simulink model "rtMotomanVR_vaja7"  (R2019b)
settings: Solver=FixedStepDiscrete  StartTime=0.0  StopTime=30  FixedStep=dT  RelTol=1e-3  EnableMultiTasking=on
values from neighbouring files (symbols this model uses):
  dT = 1/500    (= 0.002)    [initVR.m]    (also in trajectory.m = 0.00025)
  fbGain = 20    [initVR.m]    (also in trajectory.m)
  q0 = [0 0 0 0 90 0]'*pi/180    [initVR.m]    (also in trajectory.m)
undefined symbols (not defined in the file or in its folder): DiscIntNeverNeededParam, q2ZYXeul
libraries: simulink x2, xpcutilitieslib x2, dspnetwork x2, dspinverses x1
Description:
  | Real-Time Van der Pol Simulation
  | 
  | This demonstration shows a real-time version of the Simulink Van der Pol
  | simulation demo. This model does not need any external signals, so it does
  | not need any data acquisition hardware or driver. This makes the model ideal
  | for first experiments with Real-Time Windows Target, without need to
  | worry about proper I/O hardware configuration.
  | 
  | How to run this demo:
  | 
  |   1. Build the model using Tools -> Real-Time Workshop -> Build Model.
  |   2. Connect to the real-time code using Simulation -> Connect to target.
  |   3. Start the real-time execution using Simulation -> Start real-time code.
settings Model: EnablePacing=on  Creator=Houska  LastModifiedBy=student
settings DataIOCC: LimitDataPoints=on  SaveFormat=Array  SignalLoggingSaveFormat=ModelDataLogs  SaveOutput=off  SaveTime=off  ReturnWorkspaceOutputs=off  SignalLoggingName=logsOut
settings OptimizationCC: ExpressionDepthLimit=2147483647  InitFltsAndDblsToZero=on  LifeSpan=inf
settings DebuggingCC: SaveWithParameterizedLinksMsg=none  UnderspecifiedInitializationDetection=Classic  MergeDetectMultiDrivingBlocksExec=none  SignalResolutionControl=TryResolveAllWithWarning  MultiTaskDSMMsg=warning  MultiTaskCondExecSysMsg=none  FcnCallInpInsideContextMsg=warning  StateNameClashWarn=warning  SFUnexpectedBacktrackingDiag=warning  SFNoUnconditionalDefaultTransitionDiag=warning  SFExecutionAtInitializationDiag=none  ArithmeticOperatorsInVariantConditions=warning
settings HardwareCC: ProdBitPerPointer=32  ProdBitPerSizeT=32  ProdBitPerPtrDiffT=32  ProdLargestAtomicFloat=None  ProdWordSize=32  ProdHWDeviceType=32-bit Real-Time Windows Target
settings ModelReferenceCC: PropagateSignalLabelsOutOfModel=off
settings SFSimCC: SimUseLocalCustomCode=off  SimParseCustomCode=off  CustomCodeUndefinedFunction=UseInterfaceOnly
settings RTWCC: Description=Real-Time Windows Target  SystemTargetFile=rtwin.tlc  TemplateMakefile=rtwin.tmf  RTWUseLocalCustomCode=off
settings CodeAppCC: StateflowObjectComments=on
settings TargetCC: TargetFcnLib=ansi_tfl_tmw.mat  ModelReferenceCompliant=off  CompOptLevelCompliant=off  PreserveStateflowLocalDataDimensions=off
settings ConfigComp: CovMetricSettings=dw  CovHtmlReporting=on  CovSaveCumulativeToWorkspaceVar=on  CovSaveSingleToWorkspaceVar=on  CovExternalEMLEnable=off

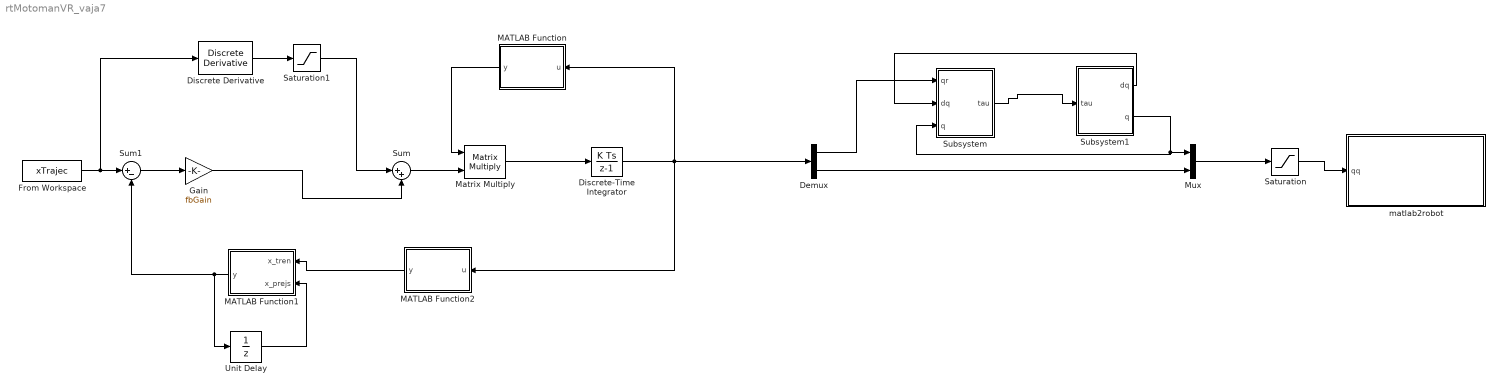
== system rtMotomanVR_vaja7 ==
  Demux : Demux  Outputs=2
  Discrete Derivative : simulink/Discrete/Discrete Derivative  gainval=1.0  ICPrevScaledInput=0.0  OutMin=[]  OutMax=[]  OutDataType=fixdt(1, 16)  OutScaling=2^-10  DoSatur=off
  Discrete-Time Integrator : DiscreteIntegrator  InitialCondition=q0  SampleTime=dT  ICPrevOutput=DiscIntNeverNeededParam  ICPrevScaledInput=DiscIntNeverNeededParam
  From Workspace : FromWorkspace  VariableName=xTrajec  SampleTime=0
  Gain : Gain  Gain=fbGain
  MATLAB Function : MATLAB Function  TreatAsAtomicUnit=on
  MATLAB Function1 : MATLAB Function  TreatAsAtomicUnit=on
  MATLAB Function2 : MATLAB Function  TreatAsAtomicUnit=on
  Matrix Multiply : Product  Multiplication=Matrix(*)
  Mux : Mux  Inputs=2
  Saturation : Saturate  UpperLimit=([94.5, 75, 45, 160, 120 180]-5)*pi/180  LowerLimit=([-94.5, -40, -75, -160, -120, -180]+5)*pi/180
  Saturation1 : Saturate
  Subsystem : Subsystem
  Subsystem1 : Subsystem
  Sum : Sum  Inputs=|++
  Sum1 : Sum  Inputs=|+-
  Unit Delay : UnitDelay  InitialCondition=q2ZYXeul(q0)  SampleTime=-1  HasFrameUpgradeWarning=on
  matlab2robot : Subsystem  mask{selUDP=Simulacija, slrt_ip='192.168.65.250', slrt_port=55555, sampleTime=dT}
      mask prompts: selUDP "Izvajanje programa:"; slrt_ip "Simulink Real Time IP:"; slrt_port "Simulink Real Time Port:"; sampleTime "Vzorcni cas:"
      mask init:
      | switch selUDP
      |     case 1
      |         enSim = 1;
      |         enRob = 0;
      |     case 2
      |         enSim = 0;
      |         enRob = 1;
      |     otherwise
      |         enSim = 0;
      |         enRob = 0;
      | end
      mask TypeOptions selUDP: Simulacija | Robot
  wires:
  Saturation/1 -> matlab2robot/1(qq)
  Unit Delay/1 -> MATLAB Function1/2(x_prejs)
  From Workspace/1 -> Discrete Derivative/1, Sum1/1
  Gain/1 -> Sum/2
  MATLAB Function1/1(y) -> Unit Delay/1, Sum1/2
  MATLAB Function/1(y) -> Matrix Multiply/1
  Sum1/1 -> Gain/1
  MATLAB Function2/1(y) -> MATLAB Function1/1(x_tren)
  Discrete-Time Integrator/1 -> MATLAB Function/1(u), Demux/1, MATLAB Function2/1(u)
  Saturation1/1 -> Sum/1
  Discrete Derivative/1 -> Saturation1/1
  Sum/1 -> Matrix Multiply/2
  Matrix Multiply/1 -> Discrete-Time Integrator/1
  Mux/1 -> Saturation/1
  Demux/1 -> Subsystem/1(qr)
  Subsystem1/2(q) -> Subsystem/3(q), Mux/1
  Subsystem1/1(dq) -> Subsystem/2("dq ")
  Demux/2 -> Mux/2
  Subsystem/1("tau ") -> Subsystem1/1(tau)

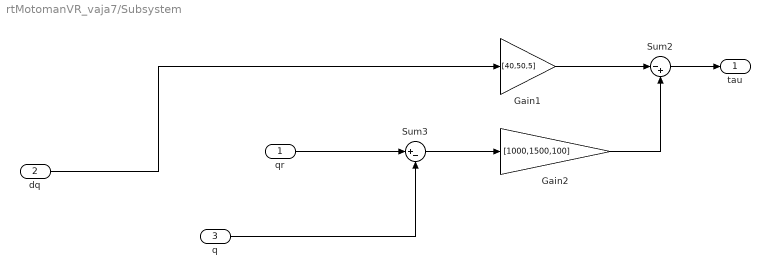
== system rtMotomanVR_vaja7/Subsystem ==
  qr : Inport
  "dq " : Inport  Port=2
  q : Inport  Port=3
  Gain1 : Gain  Gain=[40,50,5]
  Gain2 : Gain  Gain=[1000,1500,100]
  Sum2 : Sum  Inputs=|-+
  Sum3 : Sum  Inputs=|+-
  "tau " : Outport
  wires:
  Sum3/1 -> Gain2/1
  qr/1 -> Sum3/1
  Gain2/1 -> Sum2/2
  Gain1/1 -> Sum2/1
  Sum2/1 -> "tau "/1
  q/1 -> Sum3/2
  "dq "/1 -> Gain1/1

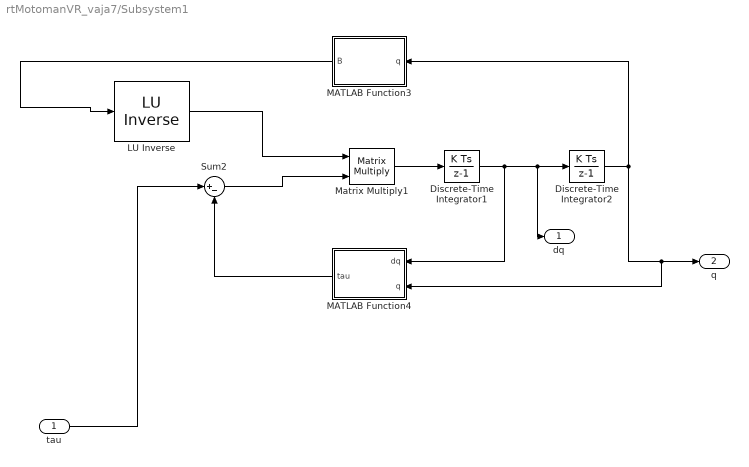
== system rtMotomanVR_vaja7/Subsystem1 ==
  tau : Inport
  " LU Inverse" : dspinverses/ LU Inverse
      settings: SourceProductName=DSP System Toolbox
  Discrete-Time Integrator1 : DiscreteIntegrator  InitialCondition=[0 0 0]  SampleTime=dT  ICPrevOutput=DiscIntNeverNeededParam  ICPrevScaledInput=DiscIntNeverNeededParam
  Discrete-Time Integrator2 : DiscreteIntegrator  InitialCondition=q0(1:3)  SampleTime=dT  ICPrevOutput=DiscIntNeverNeededParam  ICPrevScaledInput=DiscIntNeverNeededParam
  MATLAB Function3 : MATLAB Function  TreatAsAtomicUnit=on
  MATLAB Function4 : MATLAB Function  TreatAsAtomicUnit=on
  Matrix Multiply1 : Product  Multiplication=Matrix(*)
  Sum2 : Sum  Inputs=|+-
  dq : Outport
  q : Outport  Port=2
  wires:
  Sum2/1 -> Matrix Multiply1/2
  " LU Inverse"/1 -> Matrix Multiply1/1
  MATLAB Function4/1(tau) -> Sum2/2
  MATLAB Function3/1(B) -> " LU Inverse"/1
  Matrix Multiply1/1 -> Discrete-Time Integrator1/1
  tau/1 -> Sum2/1
  Discrete-Time Integrator1/1 -> dq/1, Discrete-Time Integrator2/1, MATLAB Function4/1(dq)
  Discrete-Time Integrator2/1 -> MATLAB Function4/2(q), q/1, MATLAB Function3/1(q)

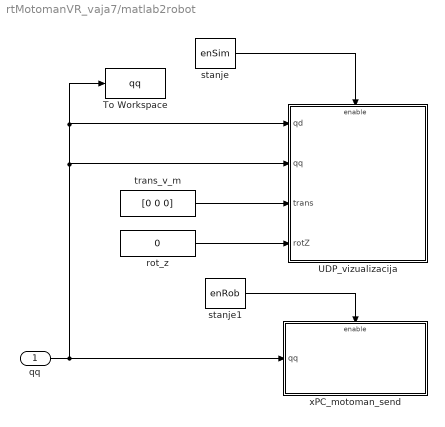
== system rtMotomanVR_vaja7/matlab2robot ==
  qq : Inport
  To Workspace : ToWorkspace  VariableName=qq  SampleTime=-1
  UDP_vizualizacija : Subsystem
  rot_z : Constant  Value=0
  stanje : Constant  Value=enSim  SampleTime=dT
  stanje1 : Constant  Value=enRob  SampleTime=dT
  trans_v_m : Constant  Value=[0 0 0]
  xPC_motoman_send : Subsystem  mask{IDSeje=rand(1), GetReady=1, slrt_ip1=slrt_ip, slrt_port1=slrt_port}
      mask prompts: IDSeje "IDSeje Function"; GetReady "GetReady Function"; slrt_ip1 "xPC Target IP"; slrt_port1 "xPC Target port"
      mask init:
      | %set_param([gcb,'/Send'],'remoteURL',slrt_ip1);
      | %set_param([gcb,'/Send'],'remotePort',num2str(slrt_port1));
      mask Callback slrt_port1: % set_param([gcb,'/Send'],'ipPort',slrt_port)
  wires:
  stanje/1 -> UDP_vizualizacija/Enable
  rot_z/1 -> UDP_vizualizacija/4(rotZ)
  trans_v_m/1 -> UDP_vizualizacija/3(trans)
  qq/1 -> To Workspace/1, UDP_vizualizacija/1(qd), UDP_vizualizacija/2(qq), xPC_motoman_send/1(qq)
  stanje1/1 -> xPC_motoman_send/Enable

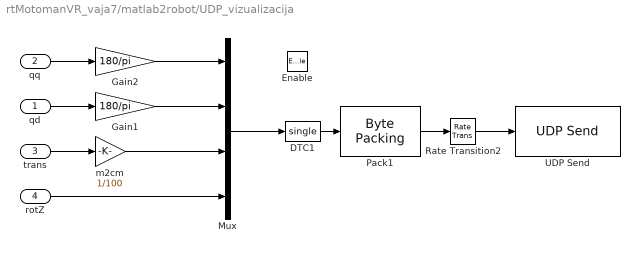
== system rtMotomanVR_vaja7/matlab2robot/UDP_vizualizacija ==
  qd : Inport
  qq : Inport  Port=2
  trans : Inport  Port=3
  rotZ : Inport  Port=4
  Enable : EnablePort  StatesWhenEnabling=reset
  DTC1 : DataTypeConversion  OutDataTypeStr=single
  Gain1 : Gain  Gain=180/pi
  Gain2 : Gain  Gain=180/pi
  Mux : Mux
  Pack1 : xpcutilitieslib/Byte Packing   MaskPackedDataType=uint8  MaskUnpackedDataTypes={'single'}  MaskAlignment=1
  Rate Transition2 : RateTransition
  UDP Send : dspnetwork/UDP Send  remoteURL='127.0.0.1'  remotePort=25300  localURL='0.0.0.0'  localPortSource=Automatically determine  localPort=-1  sampletime=-1  blockPlatform=[]  separateLengthPort=0
      settings: SourceProductName=Simulink
  m2cm : Gain  Gain=1/100
  wires:
  trans/1 -> m2cm/1
  Mux/1 -> DTC1/1
  m2cm/1 -> Mux/3
  rotZ/1 -> Mux/4
  qq/1 -> Gain2/1
  qd/1 -> Gain1/1
  Gain2/1 -> Mux/1
  Gain1/1 -> Mux/2
  Pack1/1 -> Rate Transition2/1
  Rate Transition2/1 -> UDP Send/1
  DTC1/1 -> Pack1/1

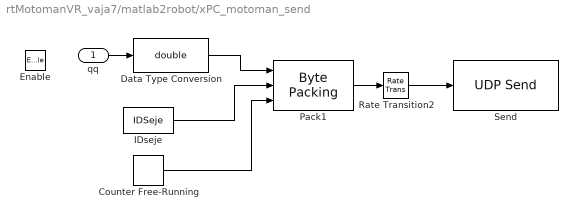
== system rtMotomanVR_vaja7/matlab2robot/xPC_motoman_send ==
  qq : Inport
  Enable : EnablePort  StatesWhenEnabling=reset
  Counter Free-Running : simulink/Sources/Counter Free-Running  NumBits=16  tsamp=-1
  Data Type Conversion : DataTypeConversion  OutDataTypeStr=double  SampleTime=dT
  IDseje : Constant  Value=IDSeje  SampleTime=dT
  Pack1 : xpcutilitieslib/Byte Packing   MaskPackedDataType=uint8  MaskUnpackedDataTypes={'double','double','uint16'}  MaskAlignment=1
  Rate Transition2 : RateTransition
  Send : dspnetwork/UDP Send  remoteURL='192.168.65.250'  remotePort=55555  localURL='0.0.0.0'  localPortSource=Automatically determine  localPort=-1  sampletime=-1  blockPlatform=[]  separateLengthPort=0
      settings: SourceProductName=Simulink
  wires:
  qq/1 -> Data Type Conversion/1
  IDseje/1 -> Pack1/2
  Data Type Conversion/1 -> Pack1/1
  Counter Free-Running/1 -> Pack1/3
  Pack1/1 -> Rate Transition2/1
  Rate Transition2/1 -> Send/1

== matlab function rtMotomanVR_vaja7/MATLAB Function1 ==
  data: x_tren input; y output; x_prejs input
function y = fcn(x_tren,x_prejs )
y=x_tren;
for i = 4:6
    if abs(x_tren(i) - x_prejs(i)) >= pi
        y(i) = x_tren(i) - sign(x_tren(i) - x_prejs(i))*2*pi;
    end
end

== matlab function rtMotomanVR_vaja7/MATLAB Function ==
  data: u input; y output
function y = invJa(u)

y = ijacZYXeul(u);

== matlab function rtMotomanVR_vaja7/MATLAB Function2 ==
  data: u input; y output
function y = dirkin(u)

y = q2ZYXeul(u);

== matlab function rtMotomanVR_vaja7/Subsystem1/MATLAB Function3 ==
  data: q input; B output
function B = inertia(q)

B = inertia3(q);

== matlab function rtMotomanVR_vaja7/Subsystem1/MATLAB Function4 ==
  data: dq input; tau output; q input
function tau = tau(dq, q)

tau = tau3_q_dq(dq, q);
